simulink model "triad_activation_static_test"  (R2018b)
settings: Solver=VariableStepAuto  StartTime=0.0  StopTime=10.0  RelTol=1e-3
libraries: TriadActivation_lib x1
settings Model: Creator=Taylor  LastModifiedBy=Taylor

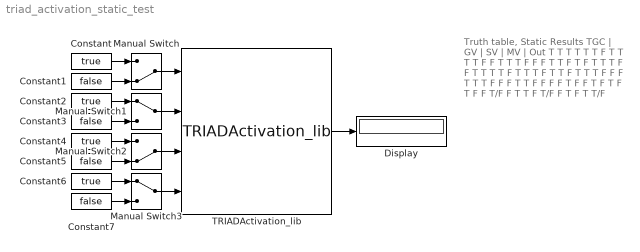
== system triad_activation_static_test ==
  note: Truth table, Static Results
      |
      | TGC | GV | SV | MV | Out
      | T T T T T
      | T F T T T
      | T F F T T
      | T F F F T
      | T F T F T
      | T T F F T
      | T T T F T
      | T T F T T
      | F T T T F
      | F F T T T
      | F F F T T
      | F F F F T
      | F F T F T
      | F T F F T/F
      | F T T F T/F
      | F T F T T/F
  Constant{,2,4,6} (4 alike) : Constant  Value=true
  Constant{1,3,5,7} (4 alike) : Constant  Value=false
  Display : Display
  Manual Switch : ManualSwitch  CurrentSetting=0
  Manual Switch1 : ManualSwitch
  Manual Switch2 : ManualSwitch  CurrentSetting=0
  Manual Switch3 : ManualSwitch
  TRIADActivation_lib : TriadActivation_lib/TRIADActivation_lib  SystemSampleTime=-1
  wires:
  TRIADActivation_lib/1 -> Display/1
  Manual Switch/1 -> TRIADActivation_lib/1
  Constant/1 -> Manual Switch/1
  Constant1/1 -> Manual Switch/2
  Constant3/1 -> Manual Switch1/2
  Constant2/1 -> Manual Switch1/1
  Manual Switch1/1 -> TRIADActivation_lib/2
  Constant4/1 -> Manual Switch2/1
  Constant5/1 -> Manual Switch2/2
  Manual Switch2/1 -> TRIADActivation_lib/3
  Constant7/1 -> Manual Switch3/2
  Constant6/1 -> Manual Switch3/1
  Manual Switch3/1 -> TRIADActivation_lib/4
